simulink model "Braccio_CtrlSimMdl"  (R2026a)
settings: Solver=ode1  StopTime=inf  FixedStep=0.01  EnableMultiTasking=on
undefined symbols (not defined in the file or in its folder): dt, efence1_coord, jnt1, jnt2, jnt3, jnt4, jnt5, Pause, Run, Shoulder
libraries: sim3dlib x16, simulink x9, Braccio_lib x8, stm32f4xxblockslib x1, robotsim3dlib x1
settings Model: STM32="{\"DigitalPortRead\":[{\"ID\":\"MotorCtrl_Demo_STM32:8\"},{\"ID\":\"DemoSetup_H755ZIQ:8\"},{\"ID\":\"DemoSetup_H755ZIQ_M7:8\"},{\"ID\":\"Aktorik_H755ZIQ_M7:8\"},{\"ID\":\"IKS4A1_H755ZIQ_M7:8\"},{\"ID\":\"BlinkModel:8\"}],\"DigitalPortWrite\":[{\"ID\":\"MotorCtrl_Demo_STM32:9\"},{\"ID\":\"MotorCtrl_Demo_STM32:26\"},{\"ID\":\"MotorCtrl_Demo_STM32:27\"},{\"ID\":\"MotorCtrl_Demo_STM32:39\"},{\"ID\":\"MotorCtrl_Demo_STM32:489\"},{\"ID\":\"MotorCtrl_Demo_STM32:493\"},{\"ID\":\"MotorCtrl_Demo_STM32:582\"},{\"ID\":\"MotorCtrl_Demo_STM32:584\"},{\"ID\":\"MotorCtrl_Demo_STM32:585\"},{\"ID\":\"MotorCtrl_Demo_STM32:586\"},{\"ID\":\"DemoSetup_H755ZIQ:9\"},{\"ID\":\"DemoSetup_H755ZIQ_M7:9\"},{\"ID\":\"Aktorik_H755ZIQ_M7:9\"},{\"ID\":\"Aktorik_H755ZIQ_M7:886\"},{\"ID\":\"Aktorik_H755ZIQ_M7:887\"},{\"ID\":\"Aktorik_H755ZIQ_M7:929\"},{\"ID\":\"Aktorik_H755ZIQ_M7:930\"},{\"ID\":\"Aktorik_H755ZIQ_M7:1123\"},{\"ID\":\"Aktorik_H755ZIQ_M7:1128\"},{\"ID\":\"Aktorik_H755ZIQ_M7:1152\"},{\"ID\":\"Aktorik_H755ZIQ_M7:1176\"},{\"ID\":\"Aktorik_H755ZIQ_M7:1222\"},{\"ID\":\"Aktorik_H755ZIQ_M7:1224\"},{\"ID\":\"Aktorik_H755ZIQ_M7:1233\"},{\"ID\":\"IKS4A1_H755ZIQ_M7:9\"},{\"ID\":\"BlinkModel:9\"},{\"ID\":\"2666\"}],\"PWMOutput\":[{\"ID\":\"MotorCtrl_Demo_STM32:23\"},{\"ID\":\"Aktorik_H755ZIQ_M7:885\"},{\"ID\":\"Aktorik_H755ZIQ_M7:988\"}],\"EncoderBlock\":[{\"ID\":\"MotorCtrl_Demo_STM32:41\"},{\"ID\":\"Aktorik_H755ZIQ_M7:1005\"}],\"AnalogInputForH7\":{\"ID\":\"Aktorik_H755ZIQ_M7:875\"},\"I2CControllerRead\":[{\"ID\":\"Aktorik_H755ZIQ_M7:1322\"},{\"ID\":\"Aktorik_H755ZIQ_M7:1414\"},{\"ID\":\"Aktorik_H755ZIQ_M7:1416\"},{\"ID\":\"Aktorik_H755ZIQ_M7:1435\"},{\"ID\":\"Aktorik_H755ZIQ_M7:1437\"},{\"ID\":\"Aktorik_H755ZIQ_M7:1438\"},{\"ID\":\"Aktorik_H755ZIQ_M7:1465\"},{\"ID\":\"Aktorik_H755ZIQ_M7:1466\"},{\"ID\":\"Aktorik_H755ZIQ_M7:1488\"},{\"ID\":\"Aktorik_H755ZIQ_M7:1489\"},{\"ID\":\"Aktorik_H755ZIQ_M7:1491\"},{\"ID\":\"Aktorik_H755ZIQ_M7:1492\"},{\"ID\":\"Aktorik_H755ZIQ_M7:1495\"},{\"ID\":\"Aktorik_H755ZIQ_M7:1496\"},{\"ID\":\"Aktorik_H755ZIQ_M7:1497\"},{\"ID\":\"Aktorik_H755ZIQ_M7:1498\"},{\"ID\":\"Aktorik_H755ZIQ_M7:1499\"},{\"ID\":\"Aktorik_H755ZIQ_M7:1500\"},{\"ID\":\"IKS4A1_H755ZIQ_M7:1435\"},{\"ID\":\"IKS4A1_H755ZIQ_M7:1437\"},{\"ID\":\"IKS4A1_H755ZIQ_M7:1438\"},{\"ID\":\"IKS4A1_H755ZIQ_M7:1414\"},{\"ID\":\"IKS4A1_H755ZIQ_M7:1416\"},{\"ID\":\"IKS4A1_H755ZIQ_M7:1495\"},{\"ID\":\"IKS4A1_H755ZIQ_M7:1496\"},{\"ID\":\"IKS4A1_H755ZIQ_M7:1497\"},{\"ID\":\"IKS4A1_H755ZIQ_M7:1498\"},{\"ID\":\"IKS4A1_H755ZIQ_M7:1499\"},{\"ID\":\"IKS4A1_H755ZIQ_M7:1500\"},{\"ID\":\"IKS4A1_H755ZIQ_M7:1465\"},{\"ID\":\"IKS4A1_H755ZIQ_M7:1466\"},{\"ID\":\"IKS4A1_H755ZIQ_M7:1488\"},{\"ID\":\"IKS4A1_H755ZIQ_M7:1489\"},{\"ID\":\"IKS4A1_H755ZIQ_M7:1491\"},{\"ID\":\"IKS4A1_H755ZIQ_M7:1492\"}],\"I2CControllerWrite\":[{\"ID\":\"Aktorik_H755ZIQ_M7:1375\"},{\"ID\":\"Aktorik_H755ZIQ_M7:1404\"},{\"ID\":\"Aktorik_H755ZIQ_M7:1452\"},{\"ID\":\"Aktorik_H755ZIQ_M7:1459\"},{\"ID\":\"Aktorik_H755ZIQ_M7:1511\"},{\"ID\":\"IKS4A1_H755ZIQ_M7:1404\"},{\"ID\":\"IKS4A1_H755ZIQ_M7:1375\"},{\"ID\":\"IKS4A1_H755ZIQ_M7:1452\"},{\"ID\":\"IKS4A1_H755ZIQ_M7:1511\"},{\"ID\":\"IKS4A1_H755ZIQ_M7:1459\"}]}"  SILPILModeSetting=veronly  ExtModeTrigDuration=10  Creator=bende  LastModifiedBy=Bender
settings OptimizationCC: PassReuseOutputArgsThreshold=0.0  MaxStackSize=256
settings HardwareCC: ProdBitPerLong=64.0  ProdHWDeviceType=Intel->x86-64 (Linux 64)  TargetBitPerPointer=64.0  TargetBitPerSizeT=64.0  TargetBitPerPtrDiffT=64.0  TargetLongLongMode=on  TargetIntDivRoundTo=Zero  TargetEndianess=LittleEndian  TargetWordSize=64.0  TargetHWDeviceType=MATLAB Host  ProdEqTarget=off
settings RTWCC: SystemTargetFile=rsim.tlc  TemplateMakefile=rsim_default_tmf  Toolchain=GNU Tools for ARM Embedded Processors  Description=Rapid Simulation Target
settings CodeAppCC: MaxIdLength=95.0
settings RSimTargetCC: ExtModeTransport=0.0  ExtModeStaticAllocSize=1000000.0  MultiwordLength=2048.0
settings SimscapeCC: SimscapeNominalValues="[{\"value\":\"1\",\"unit\":\"A\"},{\"value\":\"1\",\"unit\":\"bar\"},{\"value\":\"1\",\"unit\":\"cm^2\"},{\"value\":\"1\",\"unit\":\"cm^3/s\"},{\"value\":\"1\",\"unit\":\"kJ/kg\"},{\"value\":\"1\",\"unit\":\"kW\"},{\"value\":\"1\",\"unit\":\"l\"},{\"value\":\"1\",\"unit\":\"N\"},{\"value\":\"1\",\"unit\":\"N*m\"},{\"value\":\"1\",\"unit\":\"V\"}]"  SimscapeLogType=none  SimscapeLogDataHistory=5000.0

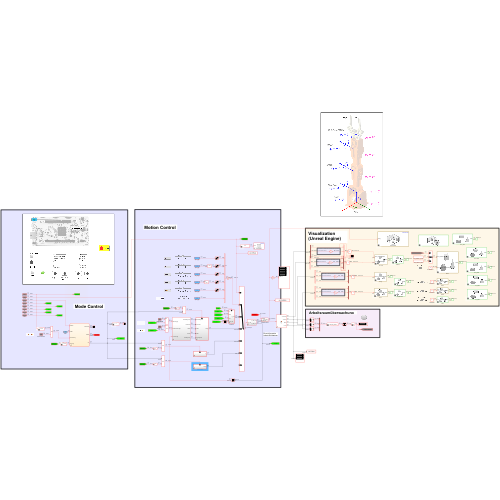
[thumbnail: Simulink's stored preview of the top-level diagram]
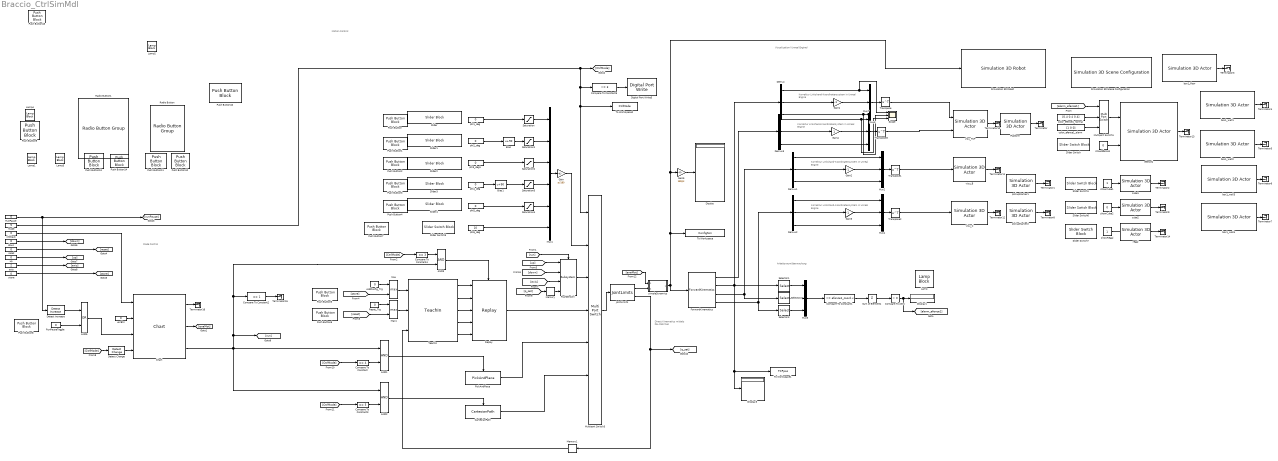
== system Braccio_CtrlSimMdl ==
  note: Korrektur Linkshand-Koordinatensystem
      | in Unreal Engine
  note: Arbeitsraumüberwachung
  note: Korrektur Linkshand-Koordinatensystem
      | in Unreal Engine
  note: Korrektur Linkshand-Koordinatensystem
      | in Unreal Engine
  note: Visualization
      | (Unreal Engine)
  note: Korrektur Linkshand-Koordinatensystem
      | in Unreal Engine
  note: Mode Control
  note: Motion Control
  note: Direct Kinematics
      | mittels DH-Matrizen
  AND1 : Logic  AllPortsSameDT=off  OutDataTypeStr=boolean
  AND2 : Logic  AllPortsSameDT=off  OutDataTypeStr=boolean
  AND3 : Logic  AllPortsSameDT=off  OutDataTypeStr=boolean
  AND5 : Logic  Operator=OR  AllPortsSameDT=off  OutDataTypeStr=boolean
  AddConfig_Trg : Constant  Value=0  SampleTime=dt
  Bias : Bias  Bias=90  SaturateOnIntegerOverflow=off
  Bias1 : Bias  Bias=90  SaturateOnIntegerOverflow=off
  CartesianPath : Braccio_lib/CartesianPath  SystemSampleTime=-1  VariantActivationTime=update diagram  EmptyChoice=off  PassThrough=off  PassThroughVariantControl=(default)  EmptyChoiceVariantControl=(default)  AllowFlexibleInterface=on  Latency=0  AutoFrameSizeCalculation=off
  Chart : Braccio_lib/Chart  SystemSampleTime=-1  VariantActivationTime=update diagram  EmptyChoice=off  PassThrough=off  PassThroughVariantControl=(default)  EmptyChoiceVariantControl=(default)  AllowFlexibleInterface=on  Latency=0  AutoFrameSizeCalculation=off
  Compare To Constant : simulink/Logic and Bit Operations/Compare To Constant  relop===  const=4  OutDataTypeStr=boolean
  Compare To Constant1 : simulink/Logic and Bit Operations/Compare To Constant  relop=<=  const=efence1_coord.x  OutDataTypeStr=boolean
  Compare To Constant2 : simulink/Logic and Bit Operations/Compare To Constant  relop===  const=1  OutDataTypeStr=boolean
  Compare To Constant3 : simulink/Logic and Bit Operations/Compare To Constant  relop===  const=5  OutDataTypeStr=boolean
  Compare To Constant4 : simulink/Logic and Bit Operations/Compare To Constant  relop===  const=3  OutDataTypeStr=boolean
  Compare To Constant5 : simulink/Logic and Bit Operations/Compare To Constant  relop=>=  const=3  OutDataTypeStr=boolean
  Compare To Zero : simulink/Logic and Bit Operations/Compare To Zero  relop=>  OutDataTypeStr=boolean
  Demux{,1..3} (4 alike) : Demux  Outputs=3
  Detect Change : simulink/Logic and Bit Operations/Detect Change  vinit=0  OutDataTypeStr=boolean
  Detect Increase : simulink/Logic and Bit Operations/Detect Increase  vinit=0.0  OutDataTypeStr=boolean
  Digital Port Write5 : stm32f4xxblockslib/Digital Port Write  PortName=GPIOD  PinNumber=7  ReadOperation=off  IOAsArray=off  EnableSimPort=off  hoistedMaskSrc=ECSoC/ECSimCodegen/Digital Port Write
      settings: LibrarySourceBlock=stm32h7xxblockslib/Digital Port Write
  Display : Display
  Display1 : Display
  Display3 : Display
  ForwardKinematics : Braccio_lib/ForwardKinematics  SystemSampleTime=-1  VariantActivationTime=update diagram  EmptyChoice=off  PassThrough=off  PassThroughVariantControl=(default)  EmptyChoiceVariantControl=(default)  AllowFlexibleInterface=on  Latency=0  AutoFrameSizeCalculation=off
  Gain : Gain  Gain=pi/180
  Gain1 : Gain  Gain=-1
  Gain2 : Gain  Gain=-1
  Gain3 : Gain  Gain=-1
  Gain4 : Gain
  Gain5 : Gain  Gain=180/pi
  JointLimits : Braccio_lib/JointLimits  SystemSampleTime=-1  VariantActivationTime=update diagram  EmptyChoice=off  PassThrough=off  PassThroughVariantControl=(default)  EmptyChoiceVariantControl=(default)  AllowFlexibleInterface=on  Latency=0  AutoFrameSizeCalculation=off
  Lamp{,1..4} (5 alike) : LampBlock  LabelPosition=Hide  DefaultColor=[192.0, 192.0, 192.0]
  Max : MinMax  Function=max  Inputs=2
  Max1 : MinMax  Function=max  Inputs=2
  Memory : Memory  InitialCondition=[0;90;0;90;0;20]*pi/180
  Memory1 : Memory  InheritSampleTime=on
  Multiport Switch1 : MultiPortSwitch  DataPortOrder=Zero-based contiguous  Inputs=2  zeroidx=on  SaturateOnIntegerOverflow=off  InputSameDT=off
  Multiport Switch3 : MultiPortSwitch  Inputs=6  SaturateOnIntegerOverflow=off  InputSameDT=off
  Mux1 : Mux  Inputs=6
  Mux{2..5,7} (5 alike) : Mux  Inputs=3
  PickAndPlace : Braccio_lib/PickAndPlace  SystemSampleTime=-1  VariantActivationTime=update diagram  EmptyChoice=off  PassThrough=off  PassThroughVariantControl=(default)  EmptyChoiceVariantControl=(default)  AllowFlexibleInterface=on  Latency=0  AutoFrameSizeCalculation=off
  Platform : sim3dlib/Simulation 3D Actor  Priority=1  ActorName=actor1_platform  ParentName=Scene Origin  Operation=Create at setup  InitScriptText=|  SampleTime=-1  Translation=[0.1 0 -0.01]  Rotation=[0 0 0]  Scale=[1 1 1]  aMode=5  ActorTag=actor1_platform  ActorType=Sim3dActor  ID=C
      | % Reserved keywords:
      | % - Actor : handle to this actor object
      | % - World : handle to the world object
      | 
      | % Examples:
      | 
      | % Create a primitive geometry (optional)
      | createShape(Actor, 'box', [0.6,0.3,0.02]);
      | 
      | % Initialize values (optional)
      | Actor.Physics = false;
      | Actor.Color = [0.4 0.4 0.4];
      | %platform = collisionBox(0.6,0.3,0.02);
      | %platform.Pose = trvec2tform([-0.1 0 -.01]);
  Push Button : PushButtonBlock  ButtonText=Reset q1  OnValue=0  ButtonType=Latch  IconOnColor=[0.0, 0.39215686274509803, 0.0]  IconOffColor=[0.0, 1.0, 0.0]  OffValue=-2.550607
  Push Button1 : PushButtonBlock  ButtonText=Reset q2  OnValue=0  ButtonType=Latch  IconOnColor=[0.0, 0.39215686274509803, 0.0]  IconOffColor=[0.0, 1.0, 0.0]  OffValue=24.257377
  Push Button10 : PushButtonBlock  ButtonText=NOTAUS  Icon=Circle  IconOnColor=[1.0, 0.0, 0.0]  IconOffColor=[1.0, 0.0, 0.0]  IconColor=On  OffValue=0.000000
  Push Button{9,11..14} (5 alike) : PushButtonBlock  Icon=Circle  IconOnColor=[0.0, 0.39215686274509803, 0.0]  IconOffColor=[0.0, 1.0, 0.0]  OffValue=0.000000
  Push Button15 : PushButtonBlock  ButtonText=USR BTN  IconOnColor=[0.0, 0.39215686274509803, 0.0]  IconOffColor=[0.0, 1.0, 0.0]  OffValue=0.000000
  Push Button2 : PushButtonBlock  ButtonText=Reset q3  OnValue=0  ButtonType=Latch  IconOnColor=[0.0, 0.39215686274509803, 0.0]  IconOffColor=[0.0, 1.0, 0.0]  OffValue=-17.636995
  Push Button3 : PushButtonBlock  ButtonText=Reset q4  OnValue=0  ButtonType=Latch  IconOnColor=[0.0, 0.39215686274509803, 0.0]  IconOffColor=[0.0, 1.0, 0.0]  OffValue=-12.105263
  Push Button4 : PushButtonBlock  ButtonText=Reset q5  OnValue=0  ButtonType=Latch  IconOnColor=[0.0, 0.39215686274509803, 0.0]  IconOffColor=[0.0, 1.0, 0.0]  OffValue=-61.435656
  Push Button5 : PushButtonBlock  ButtonText=SAVE CONFIG  IconOnColor=[0.0, 0.39215686274509803, 0.0]  IconOffColor=[0.0, 1.0, 0.0]  OffValue=0.000000
  Push Button6 : PushButtonBlock  ButtonText=RESET  IconOnColor=[0.0, 0.39215686274509803, 0.0]  IconOffColor=[0.0, 1.0, 0.0]
  Push Button7 : PushButtonBlock  ButtonText=SAVE CONFIG  IconOnColor=[0.0, 0.39215686274509803, 0.0]  IconOffColor=[0.0, 1.0, 0.0]  OffValue=0.000000
  Push Button8 : PushButtonBlock  ButtonText=Run-Pause  IconOnColor=[0.0, 0.39215686274509803, 0.0]  IconOffColor=[0.0, 1.0, 0.0]  OffValue=0.000000
  PushBtnCtrl : Braccio_lib/Subsystem  SystemSampleTime=-1  VariantActivationTime=update diagram  EmptyChoice=off  PassThrough=off  PassThroughVariantControl=(default)  EmptyChoiceVariantControl=(default)  AllowFlexibleInterface=on  Latency=0  AutoFrameSizeCalculation=off
  Radio Button : RadioButtonGroup  LabelPosition=Hide  SelectedLabel=2 - Shoulder  ButtonGroupName=Axis
  Radio Button1 : RadioButtonGroup  LabelPosition=Hide  SelectedLabel=Cartesian Control  ButtonGroupName=Mode
  Replay : Braccio_lib/Replay  SystemSampleTime=-1  VariantActivationTime=update diagram  EmptyChoice=off  PassThrough=off  PassThroughVariantControl=(default)  EmptyChoiceVariantControl=(default)  AllowFlexibleInterface=on  Latency=0  AutoFrameSizeCalculation=off
  Reset_Trg : Constant  Value=0  SampleTime=dt
  RunPause : Constant  Value=0  SampleTime=dt
  RunPauseToggle : Constant  Value=0  SampleTime=dt
  Saturation : Saturate  UpperLimit=jnt1.PositionLimits(2)*180/pi  LowerLimit=jnt1.PositionLimits(1)*180/pi
  Saturation1 : Saturate  UpperLimit=jnt2.PositionLimits(2)*180/pi  LowerLimit=jnt2.PositionLimits(1)*180/pi
  Saturation2 : Saturate  UpperLimit=jnt3.PositionLimits(2)*180/pi  LowerLimit=jnt3.PositionLimits(1)*180/pi
  Saturation3 : Saturate  UpperLimit=jnt4.PositionLimits(2)*180/pi  LowerLimit=jnt4.PositionLimits(1)*180/pi
  Saturation4 : Saturate  UpperLimit=jnt5.PositionLimits(2)*180/pi  LowerLimit=jnt5.PositionLimits(1)*180/pi
  Scope : Scope  NumInputPorts=3
      settings: ActiveDisplayYMinimum=0.35929394467848708  ActiveDisplayYMaximum=0.36634551278284788  DataLoggingVariableName=ScopeData3
  Selector1 : Selector  InputPortWidth=3  IndexOptions=Index vector (dialog)  Indices=1  OutputSizes=1
  Selector2 : Selector  InputPortWidth=3  IndexOptions=Index vector (dialog)  Indices=1  OutputSizes=1
  Selector3 : Selector  InputPortWidth=3  IndexOptions=Index vector (dialog)  Indices=1  OutputSizes=1
  Simulation 3D Robot : robotsim3dlib/Simulation 3D Robot  actorInputType=RigidBodyTree Object  RigidBodyTree=braccioRobot  ActorName=braccioRobot  existActorChekBox=off  initialTrans=[0 0 0]  initialRot=[0 0 0]  initialConfig="[0  0  0  0  0]"  EndEffector=body5  eeOffsetInpChekBox=off  eeTargetTrans=[0 0 0]  eeTargetRot=[0 0 0]  enableRegionGraspChekBox=off  regionGraspInpChekBox=off  eeTargTransDiff=[0.2 0.2 0.2]  eeTargRotDiff=[0 0 0]  enableVisualVisualization=on  enableCollisionVisualization=on  collisionGeomColor=[0 1 0]  collisionGeomTransp=0.1  inpConfEnbVal=on  inpGraspEnbVal=off  inpTransEnbVal=off  outConfEnbVal=off  outGraspEnbVal=off  outTransEnbVal=off  SampleTime=-1  ActorType=SimulinkVehicle  ID=C  aMode=6  ActorTag=braccioRobot  Mesh=RigidBodyTree
  Simulation 3D Scene Configuration : sim3dlib/Simulation 3D Scene Configuration  Priority=0  ProjectFormat=Default Scenes  SceneDesc=Empty scene  ProjectName=C:\Program Files\MATLAB\R2026a\toolbox\shared\sim3d_projects\automotive_project_windows\UE\WindowsNoEditor\VehicleSimulation.exe  ScenePath=/Game/Maps/EmptyScene  EnableOpenDRIVE=off  vehTagList={'Actor_B';'Actor_C';'Actor_TCP';'Actor_efence1';'Custom';'Scene Origin';'View1';'View2';'View3';'View4';'actor1_platform';'actor2_pickupMarker';'actor3_cube';'boxActor1';'boxActor2';'boxActor3';'boxActor4';'boxActor5';'braccioRobot'}  vehTag=View4  AttachedCameraRelativeTranslation=[0 0 0]  FreeCameraDefaultInitialTranslation=[-6, 0, 2]  AttachedCameraRelativeRotation=[0 0 0]  FreeCameraDefaultInitialRotation=[0, -15, 0]  ViewpointName=View4  FreeCameraInitialTranslation=[0.25 -0.4 0.4]  FreeCameraInitialRotation=[0 -35 110]  OpVisEn=off  Ts=0.1  EnableWindow=on  EnableRemoteAccess=off  SimulationMode=CoSimulation  SimulateUsing=Interpreted execution  EnableAnimationRecording=off  OverrideDefaultRecording=off  AnimationRecordingFileName=sim3dAnimation.mat  AnimationRecordingInterval=[0 inf]  EnableWeather=off  SunAzimuth=90  SunAltitude=40.0  EnableGeospatialSun=off  Latitude=0  Longitude=0  Date=2023-01-01  Time=10:30:00  GeoTimeZone=-5.0  SunDaylightSaving=off  wind=0  clouds=0.0  EnableVolumetricClouds=off  CloudCoverage=0  CloudAltitude=6  fog=0  rain=0  RaindropsEffect=off  SnowDensity=0  EnableGeospatial=off  TilesetSource=Earth terrain  UseTrueOrigin=off  OriginHeight=200  OriginLatitude=40.744652  OriginLongitude=-73.988864  MapStyle=Aerial  AdditionalAssetIDs=[]  UseAdvancedSunSky=off  SolarTime=11  TimeZone=-5  Day=21  Month=9  Year=2022  UseDaylightSavingTime=on  DSTStartDay=10  DSTStartMonth=3  DSTEndDay=3  DSTEndMonth=11  DSTSwitchHour=2  sensorTag=MainCamera1  sensorId=1  sensorName=MainCamera1  mountLoc=Origin  offsetFlag=off  tmountOffset=[0, 0, 0]  rmountOffset=[0, 0, 0]  HorizontalResolution=1280  VerticalResolution=720  HorizontalFOV=60  mountPoint=[0 0 0]  mountOrientation=[0 0 0]  aMode=6  ID=1  GeoTrigger=Inactive  ViewNameList={'Custom', 'View1', 'View2', 'View3', 'View4'}  ViewTranslationList={'[0 -1 0]', '[-0.5 0 0.05]', '[0 -0.5 0.05]', '[0.15 0.5 0.25]', '[0.25 -0.4 0.4]'}  ViewRotationList={'[0 0 0]', '[0 0 0]', '[0 0 90]', '[0 -5 -90]', '[0 -35 110]'}
      settings: LibrarySourceBlock=robotsim3dlib/Simulation 3D Scene Configuration
  Slider{,1..4} (5 alike) : SliderBlock  ScaleMin=-90  ScaleMax=90
  Slider Switch{,1,5..7} (5 alike) : SliderSwitchBlock
  Sum of Elements : Sum  Inputs=+
  TeachIn : Braccio_lib/TeachIn  SystemSampleTime=-1  VariantActivationTime=update diagram  EmptyChoice=off  PassThrough=off  PassThroughVariantControl=(default)  EmptyChoiceVariantControl=(default)  AllowFlexibleInterface=on  Latency=0  AutoFrameSizeCalculation=off
  Terminator{,1..16} (17 alike) : Terminator
  To Workspace : ToWorkspace  VariableName=ConfigSim  SaveFormat=Timeseries  SampleTime=-1
  To Workspace1 : ToWorkspace  VariableName=TCPpos  SaveFormat=Timeseries  SampleTime=-1
  To Workspace2 : ToWorkspace  VariableName=CtrlMode  SaveFormat=Timeseries  SampleTime=-1
  Transpose{,1..3} (4 alike) : Math  Operator=transpose
  axis : Constant  Value=2  SampleTime=dt
  box1_floor : sim3dlib/Simulation 3D Actor  Priority=1  ActorName=boxActor2  ParentName=Scene Origin  Operation=Create at setup  InitScriptText=|  SampleTime=-1  Translation=[0 -0.2 -.015]  Rotation=[0 0 0]  Scale=[1 1 1]  aMode=5  ActorTag=boxActor2  ActorType=Sim3dActor  ID=C
      | % Reserved keywords:
      | % - Actor : handle to this actor object
      | % - World : handle to the world object
      | 
      | % Examples:
      | 
      | % Create a primitive geometry (optional)
      | createShape(Actor, 'box', [0.1,0.1,0.005]);
      | 
      | % Initialize values (optional)
      | Actor.Physics = false;
      | Actor.Color = [0.4 0.4 0.4];
      | %platform = collisionBox(0.6,0.3,0.02);
      | %platform.Pose = trvec2tform([-0.1 0 -.01]);
  box1_wall1 : sim3dlib/Simulation 3D Actor  Priority=1  ActorName=boxActor3  ParentName=Scene Origin  Operation=Create at setup  InitScriptText=|  SampleTime=-1  Translation=[0 -0.15 .05-0.02]  Rotation=[0 0 0]  Scale=[1 1 1]  aMode=5  ActorTag=boxActor3  ActorType=Sim3dActor  ID=C
      | % Reserved keywords:
      | % - Actor : handle to this actor object
      | % - World : handle to the world object
      | 
      | % Examples:
      | 
      | % Create a primitive geometry (optional)
      | createShape(Actor, 'box', [0.1,0.005,0.1]);
      | 
      | % Initialize values (optional)
      | Actor.Physics = false;
      | Actor.Color = [0.4 0.4 0.4];
      | %platform = collisionBox(0.6,0.3,0.02);
      | %platform.Pose = trvec2tform([-0.1 0 -.01]);
  box1_wall2 : sim3dlib/Simulation 3D Actor  Priority=1  ActorName=boxActor4  ParentName=Scene Origin  Operation=Create at setup  InitScriptText=|  SampleTime=-1  Translation=[0 -0.25 .05-0.02]  Rotation=[0 0 0]  Scale=[1 1 1]  aMode=5  ActorTag=boxActor4  ActorType=Sim3dActor  ID=C
      | % Reserved keywords:
      | % - Actor : handle to this actor object
      | % - World : handle to the world object
      | 
      | % Examples:
      | 
      | % Create a primitive geometry (optional)
      | createShape(Actor, 'box', [0.1,0.005,0.1]);
      | 
      | % Initialize values (optional)
      | Actor.Physics = false;
      | Actor.Color = [0.4 0.4 0.4];
      | %platform = collisionBox(0.6,0.3,0.02);
      | %platform.Pose = trvec2tform([-0.1 0 -.01]);
  box1_wall3 : sim3dlib/Simulation 3D Actor  Priority=1  ActorName=boxActor5  ParentName=Scene Origin  Operation=Create at setup  InitScriptText=|  SampleTime=-1  Translation=[0.05 -0.2 0.05-0.02]  Rotation=[0 0 0]  Scale=[1 1 1]  aMode=5  ActorTag=boxActor5  ActorType=Sim3dActor  ID=C
      | % Reserved keywords:
      | % - Actor : handle to this actor object
      | % - World : handle to the world object
      | 
      | % Examples:
      | 
      | % Create a primitive geometry (optional)
      | createShape(Actor, 'box', [0.005,0.1,0.1]);
      | 
      | % Initialize values (optional)
      | Actor.Physics = false;
      | Actor.Color = [0.4 0.4 0.4];
      | %platform = collisionBox(0.6,0.3,0.02);
      | %platform.Pose = trvec2tform([-0.1 0 -.01]);
  box1_wall4 : sim3dlib/Simulation 3D Actor  Priority=1  ActorName=boxActor1  ParentName=Scene Origin  Operation=Create at setup  InitScriptText=|  SampleTime=-1  Translation=[-0.05 -0.2 0.05-0.02]  Rotation=[0 0 0]  Scale=[1 1 1]  aMode=5  ActorTag=boxActor1  ActorType=Sim3dActor  ID=C
      | % Reserved keywords:
      | % - Actor : handle to this actor object
      | % - World : handle to the world object
      | 
      | % Examples:
      | 
      | % Create a primitive geometry (optional)
      | createShape(Actor, 'box', [0.005,0.1,0.1]);
      | 
      | % Initialize values (optional)
      | Actor.Physics = false;
      | Actor.Color = [0.4 0.4 0.4];
      | %platform = collisionBox(0.6,0.3,0.02);
      | %platform.Pose = trvec2tform([-0.1 0 -.01]);
  color_efence1_alarm : Constant  Value=[1 0 0]  SampleTime=0.01
  color_efence1_normal : Constant  Value=[0.4 0.4 0.4]  SampleTime=0.01
  cube1 : sim3dlib/Simulation 3D Actor  Priority=1  ActorName=actor_cube1  ParentName=Scene Origin  Operation=Create at setup  InitScriptText=|  SampleTime=-1  Translation=[0.25 0 0.02/2]  Rotation=[0 0 0]  Scale=[1 1 1]  InputsText=actor_cube1.Transparency  aMode=5  ActorTag=actor_cube1  ActorType=Sim3dActor  ID=C
      | % Reserved keywords:
      | % - Actor : handle to this actor object
      | % - World : handle to the world object
      | 
      | % Examples:
      | 
      | % Create a primitive geometry (optional)
      | createShape(Actor, 'box', [0.02,0.02,0.02]);
      | 
      | % Initialize values (optional)
      | Actor.Physics = false;
      | Actor.Color = [0 0 1];
      | %platform = collisionBox(0.6,0.3,0.02);
      | %platform.Pose = trvec2tform([-0.1 0 -.01]);
  cube2 : sim3dlib/Simulation 3D Actor  Priority=1  ActorName=actor_cube2  ParentName=Scene Origin  Operation=Create at setup  InitScriptText=|  SampleTime=-1  Translation=[0.35 0 0.02/2]  Rotation=[0 0 0]  Scale=[1 1 1]  InputsText=actor_cube2.Transparency  aMode=5  ActorTag=actor_cube2  ActorType=Sim3dActor  ID=C
      | % Reserved keywords:
      | % - Actor : handle to this actor object
      | % - World : handle to the world object
      | 
      | % Examples:
      | 
      | % Create a primitive geometry (optional)
      | createShape(Actor, 'box', [0.02,0.02,0.02]);
      | 
      | % Initialize values (optional)
      | Actor.Physics = false;
      | Actor.Color = [0 1 0];
      | %platform = collisionBox(0.6,0.3,0.02);
      | %platform.Pose = trvec2tform([-0.1 0 -.01]);
  down : Constant  Value=0  SampleTime=dt
  efence1 : sim3dlib/Simulation 3D Actor  Priority=1  ActorName=Actor_efence1  ParentName=Scene Origin  Operation=Create at setup  InitScriptText=|  SampleTime=-1  Translation=[efence1_coord.x 0 0.15]  Rotation=[0 0 0]  Scale=[1 1 1]  InputsText="Actor_efence1.Color        Actor_efence1.Transparency"  aMode=5  ActorTag=Actor_efence1  ActorType=Sim3dActor  ID=C
      | % Reserved keywords:
      | % - Actor : handle to this actor object
      | % - World : handle to the world object
      | 
      | % Examples:
      | 
      | % Create a primitive geometry (optional)
      | createShape(Actor, 'box', [0.002,0.3,0.3]);
      | 
      | % Initialize values (optional)
      | Actor.Physics = false;
      | Actor.Color = [0.4 0.4 0.4];
      | Actor.Transparency = 0.4;
      | %platform = collisionBox(0.6,0.3,0.02);
      | %platform.Pose = trvec2tform([-0.1 0 -.01]);
  mode : Constant  Value=5  SampleTime=dt
  phi1_deg : Constant  Value=0  SampleTime=0.01
  phi2_deg : Constant  Value=0  VectorParams1D=off  SampleTime=0.01
  phi3_deg1 : Constant  Value=0  SampleTime=0.01
  phi4_deg : Constant  Value=0  SampleTime=0.01
  phi5_deg : Constant  Value=0  SampleTime=0.01
  phi6_deg : Constant  Value=10  SampleTime=0.01
  pickupMarker1 : sim3dlib/Simulation 3D Actor  Priority=1  ActorName=actor2_pickupMarker  ParentName=Scene Origin  Operation=Create at setup  InitScriptText=|  SampleTime=-1  Translation=[0.25 0 -.005]  Rotation=[0 0 0]  Scale=[1 1 1]  aMode=5  ActorTag=actor2_pickupMarker  ActorType=Sim3dActor  ID=C
      | % Reserved keywords:
      | % - Actor : handle to this actor object
      | % - World : handle to the world object
      | 
      | % Examples:
      | 
      | % Create a primitive geometry (optional)
      | createShape(Actor, 'box', [0.025,0.025,0.012]);
      | 
      | % Initialize values (optional)
      | Actor.Physics = false;
      | Actor.Color = [0.3 0.3 0.3];
      | %platform = collisionBox(0.6,0.3,0.02);
      | %platform.Pose = trvec2tform([-0.1 0 -.01]);
  pickupMarker2 : sim3dlib/Simulation 3D Actor  Priority=1  ActorName=Sim3dActor1  ParentName=Scene Origin  Operation=Create at setup  InitScriptText=|  SampleTime=-1  Translation=[0.35 0 -.005]  Rotation=[0 0 0]  Scale=[1 1 1]  aMode=5  ActorTag=Sim3dActor1  ActorType=Sim3dActor  ID=1
      | % Reserved keywords:
      | % - Actor : handle to this actor object
      | % - World : handle to the world object
      | 
      | % Examples:
      | 
      | % Create a primitive geometry (optional)
      | createShape(Actor, 'box', [0.025,0.025,0.012]);
      | 
      | % Initialize values (optional)
      | Actor.Physics = false;
      | Actor.Color = [0.3 0.3 0.3];
      | %platform = collisionBox(0.6,0.3,0.02);
      | %platform.Pose = trvec2tform([-0.1 0 -.01]);
  regal : sim3dlib/Simulation 3D Actor  Priority=1  ActorName=actor_regal  ParentName=Scene Origin  Operation=Create at setup  InitScriptText=|  SampleTime=-1  Translation=[0.4 0 0.05]  Rotation=[0 0 0]  Scale=[1 1 1]  InputsText=actor_regal.Transparency  aMode=5  ActorTag=actor_regal  ActorType=Sim3dActor  ID=C
      | % Reserved keywords:
      | % - Actor : handle to this actor object
      | % - World : handle to the world object
      | 
      | % Examples:
      | 
      | % Create a primitive geometry (optional)
      | createShape(Actor, 'box', [0.04,0.06,0.1]);
      | 
      | % Initialize values (optional)
      | Actor.Physics = false;
      | Actor.Color = [0.3 0.3 0.3];
      | %platform = collisionBox(0.6,0.3,0.02);
      | %platform.Pose = trvec2tform([-0.1 0 -.01]);
  reset : Constant  Value=0  SampleTime=dt
  showCube1 : Constant  SampleTime=0.01
  showCube2 : Constant  Value=0  SampleTime=0.01
  showEfence1 : Constant  Value=0  SampleTime=0.01
  showRegal : Constant  SampleTime=0.01
  simpleDynamics : Subsystem
  store : Constant  Value=0  SampleTime=dt
  up : Constant  Value=0  SampleTime=dt
  usrBtn : Constant  Value=0  SampleTime=dt
  visu_B : sim3dlib/Simulation 3D Actor  Priority=1  ActorName=Actor_B  ParentName=Scene Origin  Operation=Create at setup  InitScriptText=|  SampleTime=-1  Translation=box_trans  Rotation=[0 0 0]  Scale=[1 1 1]  InputsText=Actor_B.Translation  aMode=5  ActorTag=Actor_B  ActorType=Sim3dActor  ID=C
      | % Reserved keywords:
      | % - Actor : handle to this actor object
      | % - World : handle to the world object
      | 
      | % Examples:
      | 
      | % Create a primitive geometry (optional)
      | createShape(Actor, 'sphere', [0.01,0.01,0.01]);
      | 
      | % Initialize values (optional)
      | Actor.Physics = false;
      | Actor.Color = [1 0 0];
      | %platform = collisionBox(0.6,0.3,0.02);
      | %platform.Pose = trvec2tform([-0.1 0 -.01]);
  visu_C : sim3dlib/Simulation 3D Actor  Priority=1  ActorName=Actor_C  ParentName=Scene Origin  Operation=Create at setup  InitScriptText=|  SampleTime=-1  Translation=box_trans  Rotation=[0 0 0]  Scale=[1 1 1]  InputsText=Actor_C.Translation  aMode=5  ActorTag=Actor_C  ActorType=Sim3dActor  ID=C
      | % Reserved keywords:
      | % - Actor : handle to this actor object
      | % - World : handle to the world object
      | 
      | % Examples:
      | 
      | % Create a primitive geometry (optional)
      | createShape(Actor, 'sphere', [0.01,0.01,0.01]);
      | 
      | % Initialize values (optional)
      | Actor.Physics = false;
      | Actor.Color = [1 0 0];
      | %platform = collisionBox(0.6,0.3,0.02);
      | %platform.Pose = trvec2tform([-0.1 0 -.01]);
  visu_TCP : sim3dlib/Simulation 3D Actor  Priority=1  ActorName=Actor_TCP  ParentName=Scene Origin  Operation=Create at setup  InitScriptText=|  SampleTime=-1  Translation=box_trans  Rotation=[0 0 0]  Scale=[1 1 1]  InputsText=Actor_TCP.Translation Actor_TCP.Rotation  aMode=5  ActorTag=Actor_TCP  ActorType=Sim3dActor  ID=C
      | % Reserved keywords:
      | % - Actor : handle to this actor object
      | % - World : handle to the world object
      | 
      | % Examples:
      | 
      | % Create a primitive geometry (optional)
      | createShape(Actor, 'sphere', [0.01,0.01,0.01]);
      | 
      | % Initialize values (optional)
      | Actor.Physics = false;
      | Actor.Color = [1 0 0];
      | %platform = collisionBox(0.6,0.3,0.02);
      | %platform.Pose = trvec2tform([-0.1 0 -.01]);
  xNotaus : Constant  Value=0  SampleTime=dt
  wires:
  Platform/1 -> Terminator/1
  pickupMarker1/1 -> Terminator1/1
  cube1/1 -> Terminator2/1
  box1_floor/1 -> Terminator3/1
  box1_wall1/1 -> Terminator4/1
  box1_wall2/1 -> Terminator5/1
  box1_wall3/1 -> Terminator6/1
  box1_wall4/1 -> Terminator7/1
  Mux3/1 -> Transpose/1
  Demux/3 -> Scope/2, Mux3/3
  Demux/2 -> Gain1/1
  Demux/1 -> Scope/1, Mux3/1
  Gain1/1 -> Mux3/2
  ForwardKinematics/2 -> Demux/1, Selector1/1, Display3/1, To Workspace1/1
  visu_TCP/1 -> Terminator10/1
  visu_B/1 -> Terminator11/1
  ForwardKinematics/3 -> Demux1/1, Selector2/1
  Gain2/1 -> Mux2/2
  Demux1/1 -> Mux2/1
  Demux1/2 -> Gain2/1
  Demux1/3 -> Mux2/3
  Mux2/1 -> Transpose1/1
  Mux4/1 -> Transpose2/1
  Demux2/3 -> Mux4/3
  Demux2/2 -> Gain3/1
  Gain3/1 -> Mux4/2
  ForwardKinematics/4 -> Demux2/1, Selector3/1
  visu_C/1 -> Terminator12/1
  Demux2/1 -> Mux4/1
  efence1/1 -> Terminator13/1
  Selector1/1 -> Mux5/1
  Selector2/1 -> Mux5/2
  Selector3/1 -> Mux5/3
  Mux5/1 -> Compare To Constant1/1
  Compare To Constant1/1 -> Sum of Elements/1
  Sum of Elements/1 -> Compare To Zero/1
  Compare To Zero/1 -> [alarm_efence1], Display1/1
  Multiport Switch1/1 -> efence1/1
  [alarm_efence1] -> Multiport Switch1/1
  color_efence1_normal/1 -> Multiport Switch1/2
  color_efence1_alarm/1 -> Multiport Switch1/3
  showEfence1/1 -> efence1/2
  ForwardKinematics/1 -> Demux3/1
  Gain4/1 -> Mux7/2
  Demux3/1 -> Scope/3, Mux7/1
  Demux3/2 -> Gain4/1
  Demux3/3 -> Mux7/3
  Mux7/1 -> Transpose3/1
  Transpose/1 -> visu_TCP/1
  Transpose3/1 -> visu_TCP/2
  showCube1/1 -> cube1/1
  pickupMarker2/1 -> Terminator8/1
  showCube2/1 -> cube2/1
  cube2/1 -> Terminator9/1
  regal/1 -> Terminator14/1
  showRegal/1 -> ?
  CartesianPath/1 -> Multiport Switch3/6
  AND5/1 -> Chart/3
  Chart/3 -> AND3/2, Compare To Constant2/1, [run], AND1/1, AND2/1
  usrBtn/1 -> Chart/2
  Chart/2 -> [enaMot]
  Chart/1 -> Terminator16/1
  Detect Change/1 -> Chart/4
  [CtrlMode] -> Compare To Constant3/1
  xNotaus/1 -> Chart/1
  [axis] -> PushBtnCtrl/3
  Memory/1 -> PushBtnCtrl/4
  [run] -> PushBtnCtrl/Enable
  [up] -> PushBtnCtrl/1
  [down] -> PushBtnCtrl/2
  PushBtnCtrl/1 -> Multiport Switch3/3
  [CtrlMode] -> Compare To Constant/1
  Replay/1 -> Multiport Switch3/4
  Bias/1 -> Saturation1/1
  phi4_deg/1 -> Bias1/1
  Saturation3/1 -> Mux1/4
  TeachIn/4 -> Replay/4
  phi1_deg/1 -> Saturation/1
  down/1 -> [down]
  AddConfig_Trg/1 -> Max/1
  phi6_deg/1 -> Mux1/6
  JointLimits/1 -> simpleDynamics/2(q_rad_IN)
  Saturation/1 -> Mux1/1
  phi5_deg/1 -> Saturation4/1
  Compare To Constant/1 -> AND1/2
  phi3_deg1/1 -> Saturation2/1
  AND3/1 -> Replay/Enable
  TeachIn/5 -> Replay/5
  Saturation2/1 -> Mux1/3
  AND1/1 -> PickAndPlace/Enable
  Compare To Constant3/1 -> AND2/2
  [CtrlMode] -> Compare To Constant4/1
  Saturation1/1 -> Mux1/2
  Compare To Constant2/1 -> Terminator15/1
  mode/1 -> Multiport Switch3/1, To Workspace2/1, Compare To Constant5/1, [CtrlMode]
  Multiport Switch3/1 -> JointLimits/1
  axis/1 -> [axis]
  Mux1/1 -> Gain/1
  [store] -> Max/2
  [q_set] -> Memory/1
  Gain5/1 -> Display/1
  TeachIn/1 -> Replay/1
  RunPauseToggle/1 -> AND5/2
  Reset_Trg/1 -> Max1/1
  phi2_deg/1 -> Bias/1
  up/1 -> [up]
  Max/1 -> TeachIn/1
  [CtrlMode] -> Detect Change/1
  Memory1/1 -> TeachIn/3
  Compare To Constant5/1 -> Digital Port Write5/1
  Compare To Constant4/1 -> AND3/1
  Max1/1 -> TeachIn/2
  RunPause/1 -> [runPause], Detect Increase/1
  JointLimits/2 -> [q_set], Memory1/1
  [reset] -> Max1/2
  TeachIn/2 -> Replay/2
  Gain/1 -> Multiport Switch3/2
  Detect Increase/1 -> AND5/1
  Saturation4/1 -> Mux1/5
  TeachIn/3 -> Replay/3
  Bias1/1 -> Saturation3/1
  PickAndPlace/1 -> Multiport Switch3/5
  AND2/1 -> CartesianPath/Enable
  reset/1 -> [reset]
  store/1 -> [store]
  simpleDynamics/1(q_rad_OUT) -> ForwardKinematics/1, To Workspace/1, Simulation 3D Robot/1, Gain5/1
  [enaMot] -> simpleDynamics/1(enaMot)
  Transpose1/1 -> visu_B/1
  Transpose2/1 -> visu_C/1

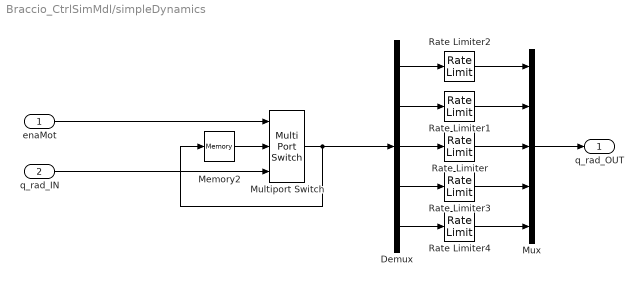
== system Braccio_CtrlSimMdl/simpleDynamics ==
  enaMot : Inport
  q_rad_IN : Inport  Port=2
  Demux : Demux  Outputs=5
  Memory2 : Memory  InitialCondition=[0;90;0;90;0]*pi/180
  Multiport Switch : MultiPortSwitch  DataPortOrder=Zero-based contiguous  Inputs=2  zeroidx=on  SaturateOnIntegerOverflow=off  InputSameDT=off
  Mux : Mux  Inputs=5
  Rate Limiter{,1..4} (5 alike) : RateLimiter  SampleTimeMode=inherited
  q_rad_OUT : Outport
  wires:
  enaMot/1 -> Multiport Switch/1
  Multiport Switch/1 -> Demux/1, Memory2/1
  Memory2/1 -> Multiport Switch/2
  q_rad_IN/1 -> Multiport Switch/3
  Mux/1 -> q_rad_OUT/1
  Demux/2 -> Rate Limiter1/1
  Demux/1 -> Rate Limiter2/1
  Rate Limiter2/1 -> Mux/1
  Rate Limiter1/1 -> Mux/2
  Demux/3 -> Rate Limiter/1
  Rate Limiter/1 -> Mux/3
  Demux/4 -> Rate Limiter3/1
  Rate Limiter3/1 -> Mux/4
  Demux/5 -> Rate Limiter4/1
  Rate Limiter4/1 -> Mux/5
